simulink model "Problem_3"  (R2020b)
settings: Solver=VariableStepAuto  StartTime=0.0  StopTime=0.05  RelTol=1e-3
settings Model: Creator=sonal  LastModifiedBy=sonal

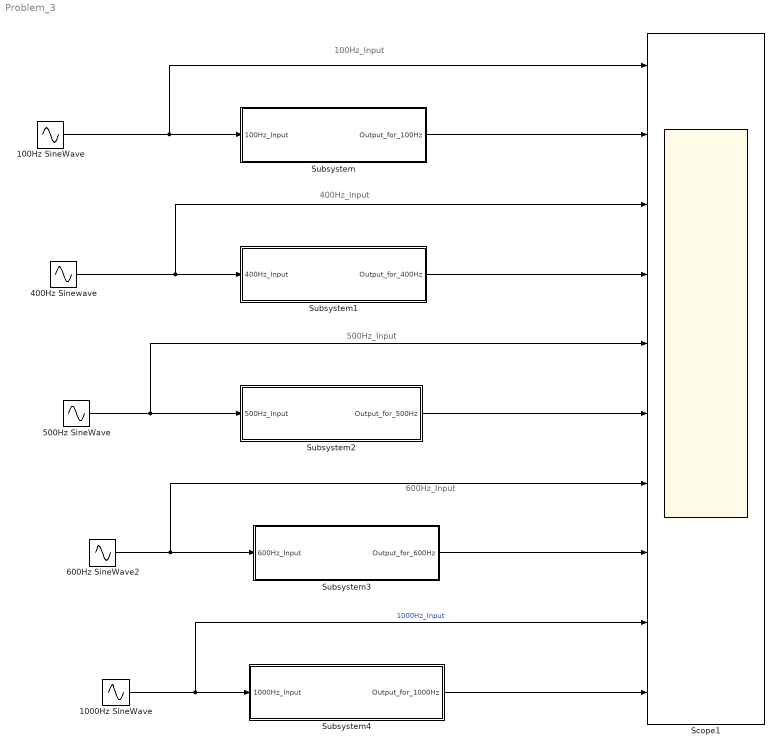
== system Problem_3 ==
  note: 100Hz_Input
  note: 500Hz_Input
  note: 400Hz_Input
  note: 600Hz_Input
  1000Hz SineWave : Sin  Frequency=2*pi*1000  SampleTime=0
  100Hz SineWave : Sin  Frequency=2*pi*100  SampleTime=0
  400Hz Sinewave : Sin  Frequency=2*pi*400  SampleTime=0
  500Hz SineWave : Sin  Frequency=2*pi*500  SampleTime=0
  600Hz SineWave2 : Sin  Frequency=2*pi*600  SampleTime=0
  Scope1 : Scope  NumInputPorts=10
  Subsystem : Subsystem
  Subsystem1 : Subsystem
  Subsystem2 : Subsystem
  Subsystem3 : Subsystem
  Subsystem4 : Subsystem
  wires:
  Subsystem/1(Output_for_100Hz) -> Scope1/2
  Subsystem1/1(Output_for_400Hz) -> Scope1/4
  Subsystem2/1(Output_for_500Hz) -> Scope1/6
  Subsystem3/1(Output_for_600Hz) -> Scope1/8
  Subsystem4/1(Output_for_1000Hz) -> Scope1/10
  100Hz SineWave/1 -> Scope1/1, Subsystem/1(100Hz_Input)
  500Hz SineWave/1 -> Scope1/5, Subsystem2/1(500Hz_Input)
  400Hz Sinewave/1 -> Scope1/3, Subsystem1/1(400Hz_Input)
  1000Hz SineWave/1 -> Scope1/9, Subsystem4/1(1000Hz_Input)  "1000Hz_Input"
  600Hz SineWave2/1 -> Scope1/7, Subsystem3/1(600Hz_Input)

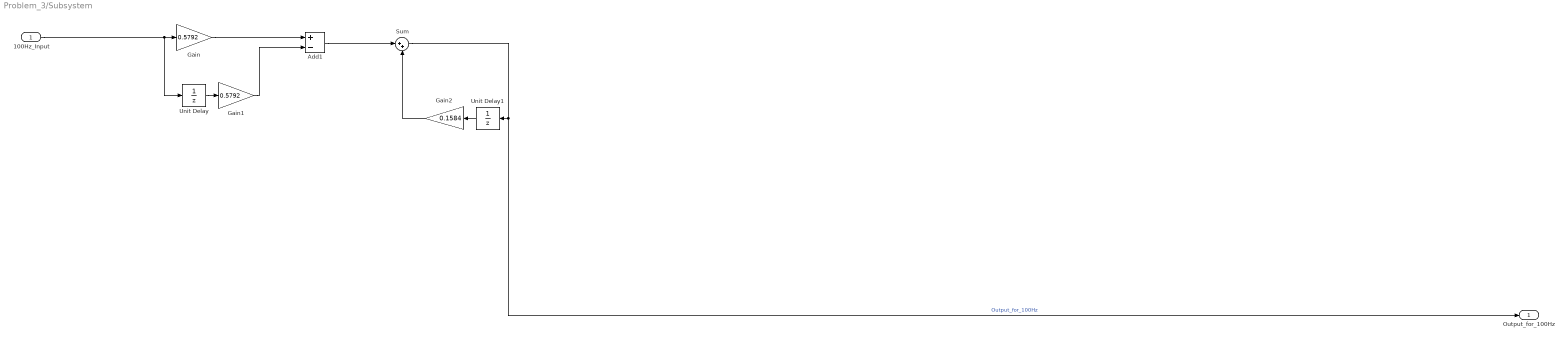
== system Problem_3/Subsystem ==
  100Hz_Input : Inport
  Add1 : Sum  Inputs=+-
  Gain : Gain  Gain=0.5792
  Gain1 : Gain  Gain=0.5792
  Gain2 : Gain  Gain=0.1584
  Sum : Sum  Inputs=|++
  Unit Delay : UnitDelay  SampleTime=-1  HasFrameUpgradeWarning=on
  Unit Delay1 : UnitDelay  SampleTime=-1  HasFrameUpgradeWarning=on
  Output_for_100Hz : Outport
  wires:
  Unit Delay/1 -> Gain1/1
  Gain2/1 -> Sum/2
  Gain/1 -> Add1/1
  Gain1/1 -> Add1/2
  100Hz_Input/1 -> Unit Delay/1, Gain/1
  Sum/1 -> Output_for_100Hz/1, Unit Delay1/1  "Output_for_100Hz"
  Unit Delay1/1 -> Gain2/1
  Add1/1 -> Sum/1

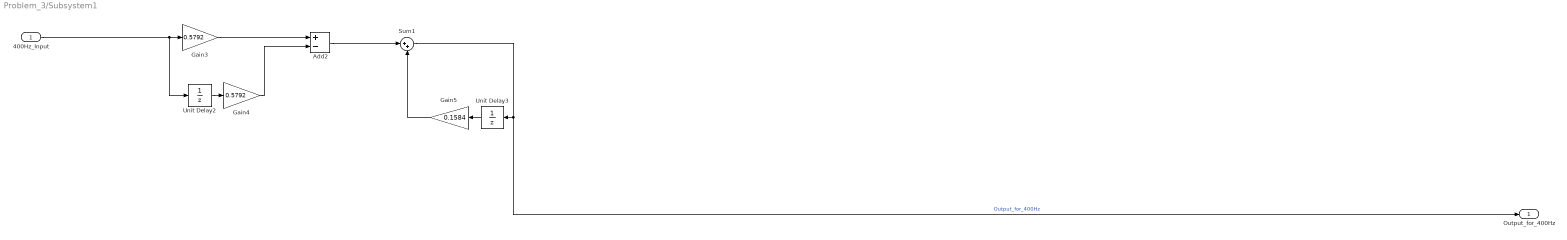
== system Problem_3/Subsystem1 ==
  400Hz_Input : Inport
  Add2 : Sum  Inputs=+-
  Gain3 : Gain  Gain=0.5792
  Gain4 : Gain  Gain=0.5792
  Gain5 : Gain  Gain=0.1584
  Sum1 : Sum  Inputs=|++
  Unit Delay2 : UnitDelay  SampleTime=-1  HasFrameUpgradeWarning=on
  Unit Delay3 : UnitDelay  SampleTime=-1  HasFrameUpgradeWarning=on
  Output_for_400Hz : Outport
  wires:
  400Hz_Input/1 -> Unit Delay2/1, Gain3/1
  Unit Delay2/1 -> Gain4/1
  Add2/1 -> Sum1/1
  Sum1/1 -> Output_for_400Hz/1, Unit Delay3/1  "Output_for_400Hz"
  Gain3/1 -> Add2/1
  Unit Delay3/1 -> Gain5/1
  Gain5/1 -> Sum1/2
  Gain4/1 -> Add2/2

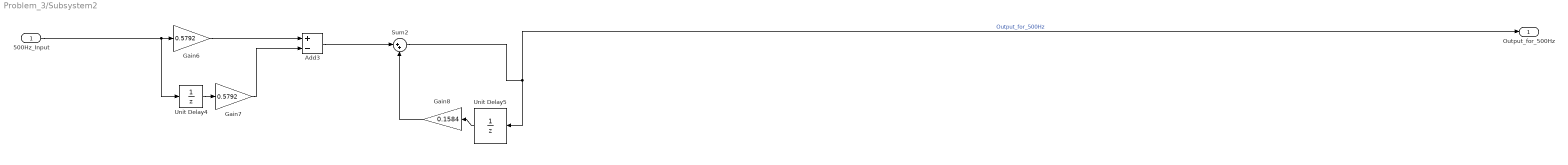
== system Problem_3/Subsystem2 ==
  500Hz_Input : Inport
  Add3 : Sum  Inputs=+-
  Gain6 : Gain  Gain=0.5792
  Gain7 : Gain  Gain=0.5792
  Gain8 : Gain  Gain=0.1584
  Sum2 : Sum  Inputs=|++
  Unit Delay4 : UnitDelay  SampleTime=-1  HasFrameUpgradeWarning=on
  Unit Delay5 : UnitDelay  SampleTime=-1  HasFrameUpgradeWarning=on
  Output_for_500Hz : Outport
  wires:
  Unit Delay5/1 -> Gain8/1
  Unit Delay4/1 -> Gain7/1
  Gain7/1 -> Add3/2
  500Hz_Input/1 -> Unit Delay4/1, Gain6/1
  Gain6/1 -> Add3/1
  Sum2/1 -> Output_for_500Hz/1, Unit Delay5/1  "Output_for_500Hz"
  Add3/1 -> Sum2/1
  Gain8/1 -> Sum2/2

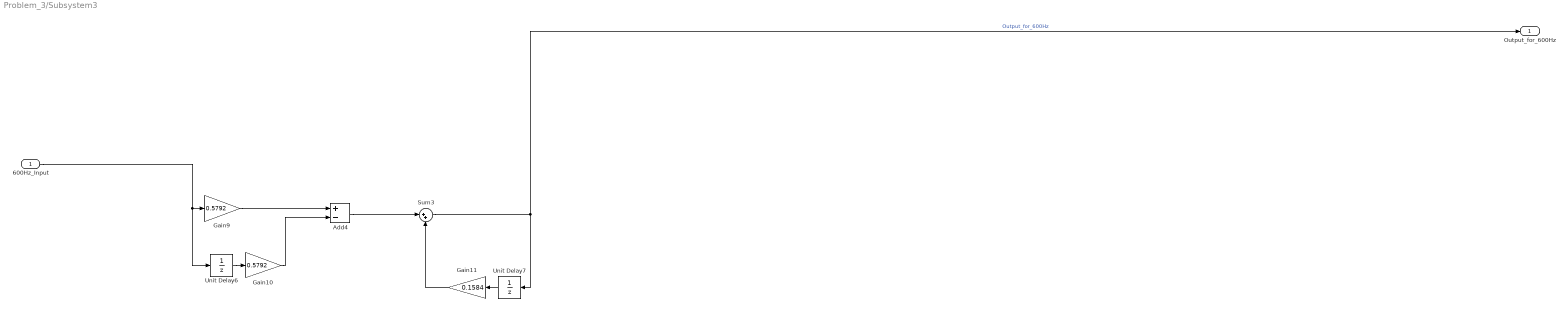
== system Problem_3/Subsystem3 ==
  600Hz_Input : Inport
  Add4 : Sum  Inputs=+-
  Gain10 : Gain  Gain=0.5792
  Gain11 : Gain  Gain=0.1584
  Gain9 : Gain  Gain=0.5792
  Sum3 : Sum  Inputs=|++
  Unit Delay6 : UnitDelay  SampleTime=-1  HasFrameUpgradeWarning=on
  Unit Delay7 : UnitDelay  SampleTime=-1  HasFrameUpgradeWarning=on
  Output_for_600Hz : Outport
  wires:
  600Hz_Input/1 -> Unit Delay6/1, Gain9/1
  Sum3/1 -> Output_for_600Hz/1, Unit Delay7/1  "Output_for_600Hz"
  Gain9/1 -> Add4/1
  Gain10/1 -> Add4/2
  Unit Delay7/1 -> Gain11/1
  Unit Delay6/1 -> Gain10/1
  Add4/1 -> Sum3/1
  Gain11/1 -> Sum3/2

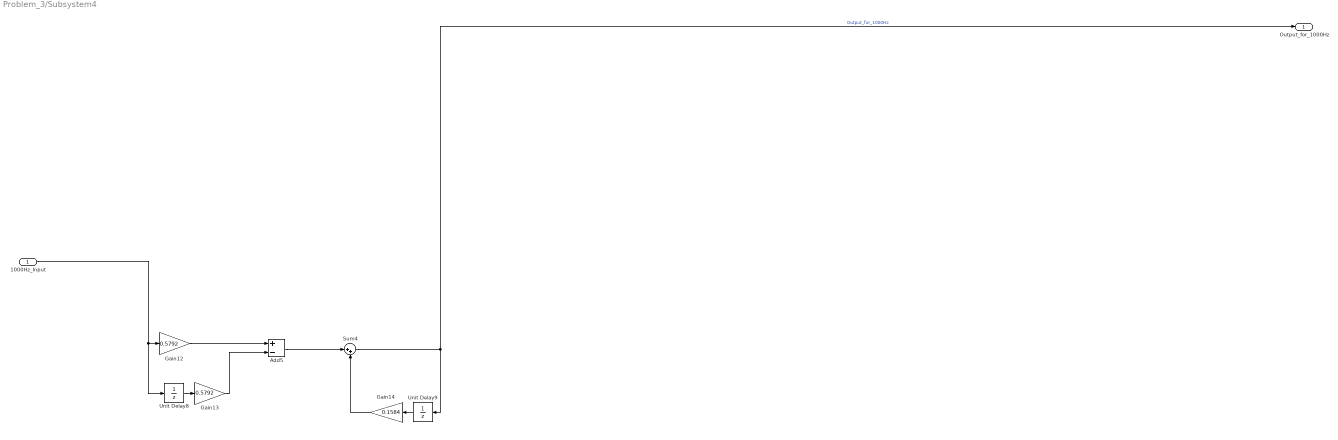
== system Problem_3/Subsystem4 ==
  1000Hz_Input : Inport
  Add5 : Sum  Inputs=+-
  Gain12 : Gain  Gain=0.5792
  Gain13 : Gain  Gain=0.5792
  Gain14 : Gain  Gain=0.1584
  Sum4 : Sum  Inputs=|++
  Unit Delay8 : UnitDelay  SampleTime=-1  HasFrameUpgradeWarning=on
  Unit Delay9 : UnitDelay  SampleTime=-1  HasFrameUpgradeWarning=on
  Output_for_1000Hz : Outport
  wires:
  Add5/1 -> Sum4/1
  1000Hz_Input/1 -> Unit Delay8/1, Gain12/1
  Gain14/1 -> Sum4/2
  Unit Delay9/1 -> Gain14/1
  Unit Delay8/1 -> Gain13/1
  Gain12/1 -> Add5/1
  Sum4/1 -> Unit Delay9/1, Output_for_1000Hz/1  "Output_for_1000Hz"
  Gain13/1 -> Add5/2
